simulink model "12_2"  (R2018b)
settings: Solver=VariableStepAuto  StartTime=0.0  StopTime=10  MaxStep=0.01  RelTol=1e-3
InitFcn:
  | Gg = [0 1; 0 0];
  | Hg = [1 0];
  | A = [0 1; 4 0];
  | B = [1; 1];
  | Bf = [2; 6];
  | C = [3 0];
  | D = 3;
  | w = 6.3/0.6;
  | %solve(s^3 + 3*w*s^2 + 3*w^2*s + w^3 == 0);
  | G_ = [0 0 -w^3; 1 0 -3*w^2; 0 1 -3*w];
  | H_ = [0 0 1];
  | G = 1;
  | A_ = [0 -G*C; zeros(2,1) A];
  | B_ = [-G*D; B];
  | 
  | M_ = sylv(-A_, G_,B_.*H_);
  | K_ = -H_*inv(M_);
  | 
  | Ke = K_(1);
  | Kx = [K_(2) K_(3)];
settings Model: Creator=kekos  LastModifiedBy=kekos

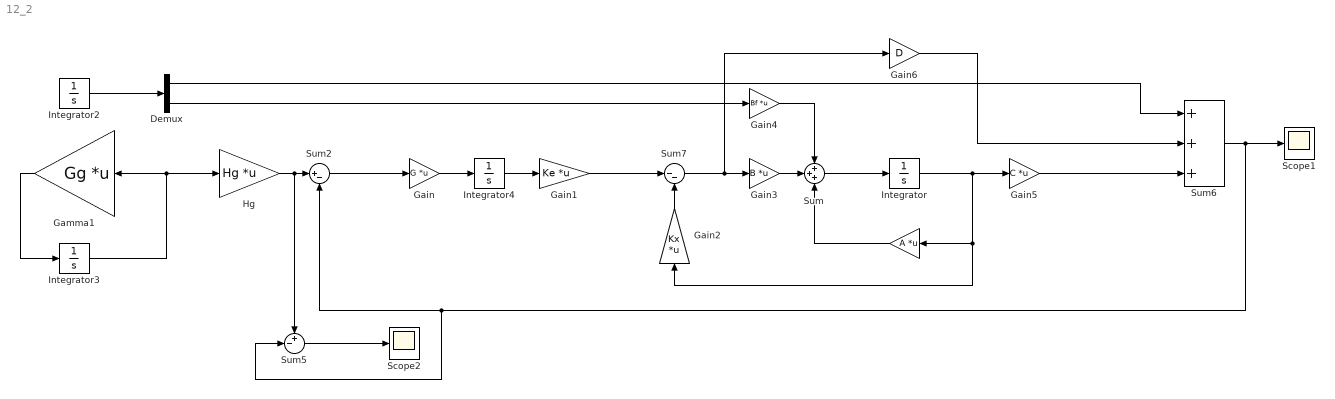
== system 12_2 ==
  " " : Gain  Gain=A  Multiplication=Matrix(K*u)
  Demux : Demux  Outputs=2
  Gain : Gain  Gain=G  Multiplication=Matrix(K*u)
  Gain1 : Gain  Gain=Ke  Multiplication=Matrix(K*u)
  Gain2 : Gain  Gain=Kx  Multiplication=Matrix(K*u)
  Gain3 : Gain  Gain=B  Multiplication=Matrix(K*u)
  Gain4 : Gain  Gain=Bf  Multiplication=Matrix(K*u)
  Gain5 : Gain  Gain=C  Multiplication=Matrix(K*u)
  Gain6 : Gain  Gain=D
  Gamma1 : Gain  Gain=Gg  Multiplication=Matrix(K*u)
  Hg : Gain  Gain=Hg  Multiplication=Matrix(K*u)
  Integrator : Integrator
  Integrator2 : Integrator  InitialCondition=[8; 6]
  Integrator3 : Integrator  InitialCondition=[0; 8]
  Integrator4 : Integrator
  Scope1 : Scope
  Scope2 : Scope
  Sum : Sum  Inputs=+++
  Sum2 : Sum  Inputs=|+-
  Sum5 : Sum  Inputs=+-|
  Sum6 : Sum  Inputs=+++
  Sum7 : Sum  Inputs=|--
  wires:
  Integrator3/1 -> Hg/1, Gamma1/1
  Gamma1/1 -> Integrator3/1
  Integrator2/1 -> Demux/1
  Gain4/1 -> Sum/1
  Hg/1 -> Sum5/1, Sum2/1
  Gain/1 -> Integrator4/1
  Integrator4/1 -> Gain1/1
  Demux/1 -> Sum6/1
  Gain6/1 -> Sum6/2
  Sum7/1 -> Gain6/1, Gain3/1
  Gain3/1 -> Sum/2
  " "/1 -> Sum/3
  Integrator/1 -> Gain5/1, " "/1, Gain2/1
  Gain1/1 -> Sum7/1
  Gain2/1 -> Sum7/2
  Gain5/1 -> Sum6/3
  Demux/2 -> Gain4/1
  Sum2/1 -> Gain/1
  Sum/1 -> Integrator/1
  Sum6/1 -> Sum5/2, Sum2/2, Scope1/1
  Sum5/1 -> Scope2/1
